simulink model "HPF0"  (R2020a)
settings: Solver=FixedStepAuto  StartTime=0.0  StopTime=10.0  FixedStep=0.2  RelTol=1e-3
settings Model: Creator=Shivam  LastModifiedBy=Shivam
settings DataIOCC: SaveOutput=off  SaveTime=off

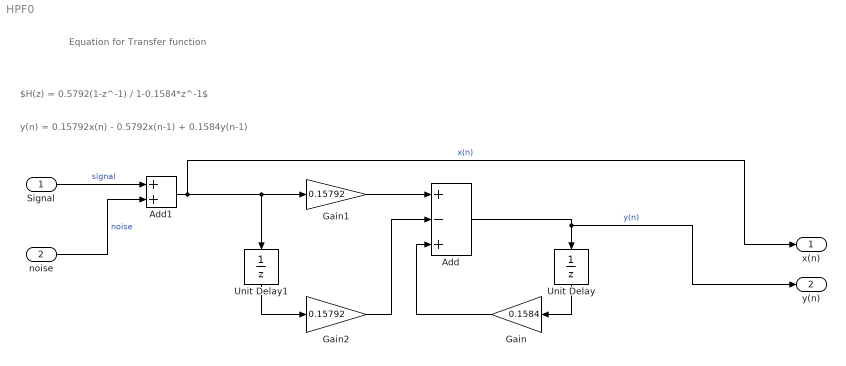
== system HPF0 ==
  note: y(n) = 0.15792x(n) - 0.5792x(n-1) + 0.1584y(n-1)
  note: $H(z) = 0.5792(1-z^-1) / 1-0.1584*z^-1$
  note: Equation for Transfer function
  Signal : Inport  OutDataTypeStr=double  PortDimensions=1  SampleTime=[0.20000000000000001,0]
  noise : Inport  Port=2  OutDataTypeStr=double  PortDimensions=1  SampleTime=[0.20000000000000001,0]
  Add : Sum  Inputs=+-+
  Add1 : Sum
  Gain : Gain  Gain=0.1584
  Gain1 : Gain  Gain=0.15792
  Gain2 : Gain  Gain=0.15792
  Unit Delay : UnitDelay  SampleTime=-1  HasFrameUpgradeWarning=on
  Unit Delay1 : UnitDelay  SampleTime=-1  HasFrameUpgradeWarning=on
  x(n) : Outport  OutDataTypeStr=double  PortDimensions=1  SampleTime=[0.20000000000000001,0]
  y(n) : Outport  Port=2  OutDataTypeStr=double  PortDimensions=1  SampleTime=[0.20000000000000001,0]
  wires:
  Add/1 -> Unit Delay/1, y(n)/1  "y(n)"
  Gain/1 -> Add/3
  Unit Delay1/1 -> Gain2/1
  noise/1 -> Add1/2  "noise"
  Unit Delay/1 -> Gain/1
  Add1/1 -> Gain1/1, Unit Delay1/1, x(n)/1  "x(n)"
  Signal/1 -> Add1/1  "signal"
  Gain2/1 -> Add/2
  Gain1/1 -> Add/1
